simulink model "aeromissile_la"  (R2019b)
settings: Solver=ode45  StartTime=0.0  StopTime=20  RelTol=1e-3  EnableMultiTasking=on
PreLoadFcn:
  | aeromissile_la_dat
values from neighbouring files (symbols this model uses):
  cy_el = 0.034000/d2r    (= 1.94805650344)    [aeromissile_la_dat.m]
  cz_el = -0.034000/d2r    (= -1.94805650344)    [aeromissile_la_dat.m]
  d_ref = 0.2286    [aeromissile_la_dat.m]
  eul_0 = [0;0;0]    [aeromissile_la_dat.m]
  fin_max = 30.0*d2r    (= 0.523598775598)    [aeromissile_la_dat.m]
  fin_min = -30.0*d2r    (= -0.523598775598)    [aeromissile_la_dat.m]
  g = 9.81    [aeromissile_la_dat.m]
  inertia = inertia_0/2    [aeromissile_la_dat.m]
  inertia_0 = diag([Ixx Iyy Izz])    [aeromissile_la_dat.m]
  l_acc = 0.5    [aeromissile_la_dat.m]
  l_ref = 0.04    [aeromissile_la_dat.m]
  len_missile = 3    [aeromissile_la_dat.m]
  mass_0 = 234.02    [aeromissile_la_dat.m]
  massf = 30    [aeromissile_la_dat.m]
  mx_el = -0.206000/d2r    (= -11.8029305797)    [aeromissile_la_dat.m]
  mx_wx = -0.5    [aeromissile_la_dat.m]
  my_el = -0.206000/d2r    (= -11.8029305797)    [aeromissile_la_dat.m]
  my_wy = -1.719    [aeromissile_la_dat.m]
  mz_el = -0.206000/d2r    (= -11.8029305797)    [aeromissile_la_dat.m]
  mz_wz = -1.719    [aeromissile_la_dat.m]
  q = 2    [aeromissile_la_dat.m]
  S_ref = 0.040877    [aeromissile_la_dat.m]
  Thrust = 10e3    (= 10000)    [aeromissile_la_dat.m]
  Vm_0 = [300;0;0]    [aeromissile_la_dat.m]
  wm_0 = [0;0;0]    [aeromissile_la_dat.m]
  x_cg = 0.555*len_missile    (= 1.665)    [aeromissile_la_dat.m]
  x_cg_0 = 0.575*len_missile    (= 1.725)    [aeromissile_la_dat.m]
  x_ref = 0.54*len_missile    (= 1.62)    [aeromissile_la_dat.m]
  xmg_0 = [0;1000;0]    [aeromissile_la_dat.m]
undefined symbols (not defined in the file or in its folder): Earth, inv_fcn, WGS84
libraries: simulink_need_slupdate x26, sharedutil x3, aerolibobsolete x2, aerolibtransform2 x2, aerolibfltsims x2, aerolibprivatev1p5 x1, vrlib x1
(part 2 of 2)

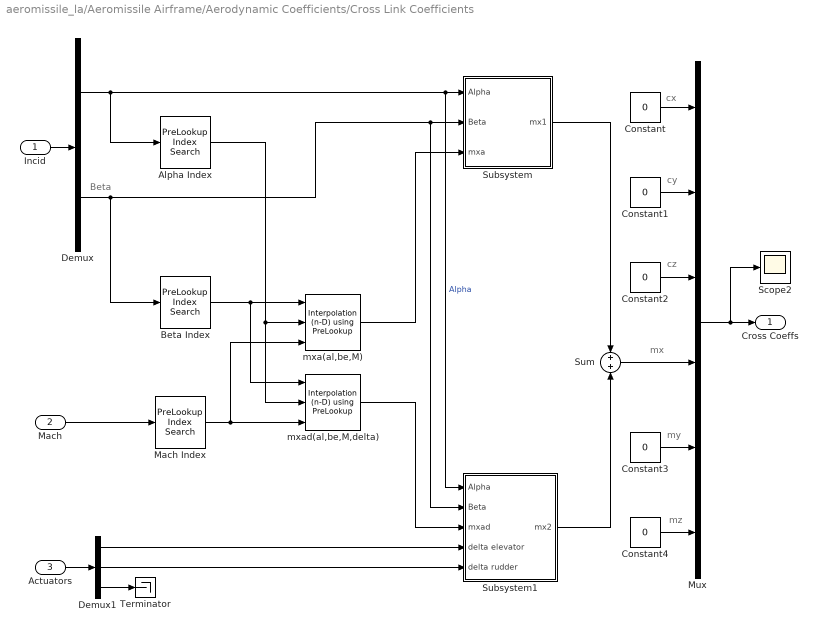
== system aeromissile_la/Aeromissile Airframe/Aerodynamic Coefficients/Cross Link Coefficients ==
  note: Beta
  note: cy
  note: cx
  note: cz
  note: mx
  note: my
  note: mz
  Incid : Inport
  Mach : Inport  Port=2
  Actuators : Inport  Port=3
  Alpha Index : simulink_need_slupdate/PreLookup Index Search  bpData=alpha_vec  searchMode=Binary Search  cacheBpFlag=on  outputFlag=off  IndexDataType=uint32  extrapMode=Linear Extrapolation  rangeErrorMode=None
      settings: SourceProductName=Simulink  SourceProductBaseCode=SL
  Beta Index : simulink_need_slupdate/PreLookup Index Search  bpData=beta_vec  searchMode=Binary Search  cacheBpFlag=on  outputFlag=off  IndexDataType=uint32  extrapMode=Linear Extrapolation  rangeErrorMode=None
      settings: SourceProductName=Simulink  SourceProductBaseCode=SL
  Constant{,1..4} (5 alike) : Constant  Value=0
  Demux : Demux  Outputs=2
  Demux1 : Demux  Outputs=3
  Mach Index : simulink_need_slupdate/PreLookup Index Search  bpData=Mach_vec  searchMode=Binary Search  cacheBpFlag=on  outputFlag=off  IndexDataType=uint32  extrapMode=Linear Extrapolation  rangeErrorMode=None
      settings: SourceProductName=Simulink  SourceProductBaseCode=SL
  Mux : Mux  Inputs=6
  Scope2 : Scope
  Subsystem : Subsystem
  Subsystem1 : Subsystem
  Sum : Sum  SaturateOnIntegerOverflow=on
  Terminator : Terminator
  mxa(al,be,M) : simulink_need_slupdate/Interpolation (n-D) using PreLookup  numDimsPopupSelect=3  explicitNumDims=2  table=mxa  interpMethod=Linear  extrapMethod=Linear  rangeErrorMode=None  NumSelectionDims=0
      settings: SourceProductName=Simulink  SourceProductBaseCode=SL
  mxad(al,be,M,delta) : simulink_need_slupdate/Interpolation (n-D) using PreLookup  numDimsPopupSelect=3  explicitNumDims=2  table=mxad  interpMethod=Linear  extrapMethod=Linear  rangeErrorMode=None  NumSelectionDims=0
      settings: SourceProductName=Simulink  SourceProductBaseCode=SL
  Cross Coeffs : Outport  InitialOutput=0
  wires:
  Mach/1 -> Mach Index/1
  Demux/1 -> Alpha Index/1, Subsystem/1(Alpha), Subsystem1/1(Alpha)  "Alpha"
  Demux/2 -> Beta Index/1, Subsystem/2(Beta), Subsystem1/2(Beta)
  Incid/1 -> Demux/1
  Constant/1 -> Mux/1
  Constant1/1 -> Mux/2
  Constant2/1 -> Mux/3
  Constant3/1 -> Mux/5
  Constant4/1 -> Mux/6
  Mux/1 -> Cross Coeffs/1, Scope2/1
  Alpha Index/1 -> mxa(al,be,M)/2, mxad(al,be,M,delta)/2
  Beta Index/1 -> mxa(al,be,M)/1, mxad(al,be,M,delta)/1
  Mach Index/1 -> mxad(al,be,M,delta)/3, mxa(al,be,M)/3
  Actuators/1 -> Demux1/1
  Demux1/1 -> Subsystem1/4(delta elevator)
  Demux1/2 -> Subsystem1/5(delta rudder)
  Demux1/3 -> Terminator/1
  Sum/1 -> Mux/4
  Subsystem/1(mx1) -> Sum/1
  mxa(al,be,M)/1 -> Subsystem/3(mxa)
  mxad(al,be,M,delta)/1 -> Subsystem1/3(mxad)
  Subsystem1/1(mx2) -> Sum/2

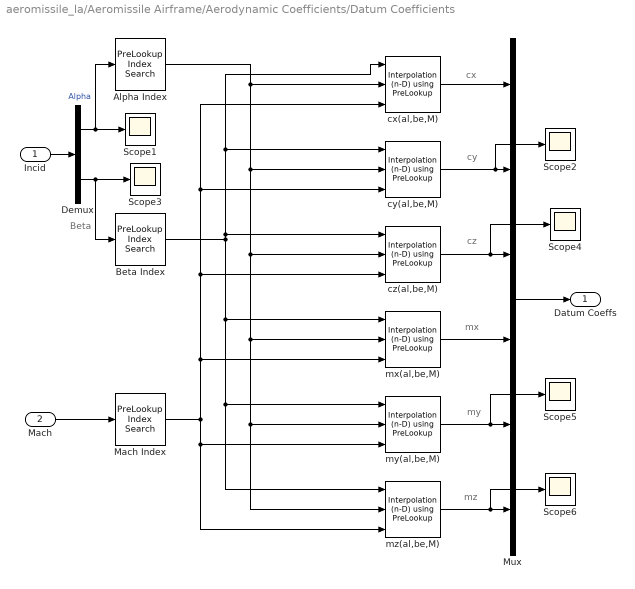
== system aeromissile_la/Aeromissile Airframe/Aerodynamic Coefficients/Datum Coefficients ==
  note: Beta
  note: cy
  note: cx
  note: cz
  note: mx
  note: my
  note: mz
  Incid : Inport
  Mach : Inport  Port=2
  Alpha Index : simulink_need_slupdate/PreLookup Index Search  bpData=alpha_vec  searchMode=Binary Search  cacheBpFlag=on  outputFlag=off  IndexDataType=uint32  extrapMode=Linear Extrapolation  rangeErrorMode=None
      settings: SourceProductName=Simulink  SourceProductBaseCode=SL
  Beta Index : simulink_need_slupdate/PreLookup Index Search  bpData=beta_vec  searchMode=Binary Search  cacheBpFlag=on  outputFlag=off  IndexDataType=uint32  extrapMode=Linear Extrapolation  rangeErrorMode=None
      settings: SourceProductName=Simulink  SourceProductBaseCode=SL
  Demux : Demux  Outputs=2
  Mach Index : simulink_need_slupdate/PreLookup Index Search  bpData=Mach_vec  searchMode=Binary Search  cacheBpFlag=on  outputFlag=off  IndexDataType=uint32  extrapMode=Linear Extrapolation  rangeErrorMode=None
      settings: SourceProductName=Simulink  SourceProductBaseCode=SL
  Mux : Mux  Inputs=6
  Scope{1..6} (6 alike) : Scope
  cx(al,be,M) : simulink_need_slupdate/Interpolation (n-D) using PreLookup  numDimsPopupSelect=3  explicitNumDims=2  table=cx  interpMethod=Linear  extrapMethod=Linear  rangeErrorMode=None  NumSelectionDims=0
      settings: SourceProductName=Simulink  SourceProductBaseCode=SL
  cy(al,be,M) : simulink_need_slupdate/Interpolation (n-D) using PreLookup  numDimsPopupSelect=3  explicitNumDims=2  table=cy  interpMethod=Linear  extrapMethod=Linear  rangeErrorMode=None  NumSelectionDims=0
      settings: SourceProductName=Simulink  SourceProductBaseCode=SL
  cz(al,be,M) : simulink_need_slupdate/Interpolation (n-D) using PreLookup  numDimsPopupSelect=3  explicitNumDims=2  table=cz  interpMethod=Linear  extrapMethod=Linear  rangeErrorMode=None  NumSelectionDims=0
      settings: SourceProductName=Simulink  SourceProductBaseCode=SL
  mx(al,be,M) : simulink_need_slupdate/Interpolation (n-D) using PreLookup  numDimsPopupSelect=3  explicitNumDims=2  table=mx  interpMethod=Linear  extrapMethod=Linear  rangeErrorMode=None  NumSelectionDims=0
      settings: SourceProductName=Simulink  SourceProductBaseCode=SL
  my(al,be,M) : simulink_need_slupdate/Interpolation (n-D) using PreLookup  numDimsPopupSelect=3  explicitNumDims=2  table=my  interpMethod=Linear  extrapMethod=Linear  rangeErrorMode=None  NumSelectionDims=0
      settings: SourceProductName=Simulink  SourceProductBaseCode=SL
  mz(al,be,M) : simulink_need_slupdate/Interpolation (n-D) using PreLookup  numDimsPopupSelect=3  explicitNumDims=2  table=mz  interpMethod=Linear  extrapMethod=Linear  rangeErrorMode=None  NumSelectionDims=0
      settings: SourceProductName=Simulink  SourceProductBaseCode=SL
  Datum Coeffs : Outport  InitialOutput=0
  wires:
  Alpha Index/1 -> my(al,be,M)/2, mz(al,be,M)/2, mx(al,be,M)/2, cz(al,be,M)/2, cy(al,be,M)/2, cx(al,be,M)/2
  Mach Index/1 -> cx(al,be,M)/3, cy(al,be,M)/3, cz(al,be,M)/3, my(al,be,M)/3, mz(al,be,M)/3, mx(al,be,M)/3
  Mach/1 -> Mach Index/1
  Beta Index/1 -> cx(al,be,M)/1, cy(al,be,M)/1, my(al,be,M)/1, mz(al,be,M)/1, mx(al,be,M)/1, cz(al,be,M)/1
  Demux/1 -> Alpha Index/1, Scope1/1  "Alpha"
  Demux/2 -> Beta Index/1, Scope3/1
  Incid/1 -> Demux/1
  cx(al,be,M)/1 -> Mux/1
  cy(al,be,M)/1 -> Mux/2, Scope2/1
  cz(al,be,M)/1 -> Mux/3, Scope4/1
  mx(al,be,M)/1 -> Mux/4
  my(al,be,M)/1 -> Mux/5, Scope5/1
  mz(al,be,M)/1 -> Mux/6, Scope6/1
  Mux/1 -> Datum Coeffs/1

== system aeromissile_la/Aeromissile Airframe/Aerodynamic Forces and Moments/Moments about Centre of Gravity ==
  Clock : Clock
  Constant1 : Constant  Value=massf
  Constant2 : Constant  Value=q
  Constant4 : Constant  Value=x_ref
  Constant5 : Constant  Value=x_cg_0
  Constant6 : Constant  Value=x_cg_0
  Constant7 : Constant  Value=x_cg
  Constant8 : Constant  Value=0
  Constant9 : Constant  Value=x_cg
  Gain1 : Gain  Gain=-1  SaturateOnIntegerOverflow=on  OutDataTypeStr=Inherit: Same as input  ParamDataTypeStr=Inherit: Same as input
  Mux : Mux  Inputs=3
  Product1 : Product  SaturateOnIntegerOverflow=on  OutDataTypeStr=Inherit: Same as first input
  Product2 : Product  Inputs=**/*  SaturateOnIntegerOverflow=on  OutDataTypeStr=Inherit: Same as first input
  Sum{2..5} (4 alike) : Sum  Inputs=|+-  SaturateOnIntegerOverflow=on
  Switch : Switch  Criteria=u2 > Threshold  SaturateOnIntegerOverflow=on
  -(x_cg-x_ref) : Outport
  tag scope: x_cg_t=global
  wires:
  Clock/1 -> Product1/2, Product2/4
  Constant1/1 -> Sum2/1, Product2/3
  Product1/1 -> Sum2/2
  Sum2/1 -> Switch/2
  Constant5/1 -> Sum3/1
  Constant6/1 -> Sum4/1
  Constant7/1 -> Sum4/2
  Product2/1 -> Sum3/2
  Sum3/1 -> Switch/1
  Constant9/1 -> Switch/3
  Switch/1 -> Sum5/1, [x_cg_t]
  Constant4/1 -> Sum5/2
  Sum5/1 -> Gain1/1
  Gain1/1 -> Mux/1
  Mux/1 -> -(x_cg-x_ref)/1
  Constant8/1 -> Mux/3, Mux/2
  Constant2/1 -> Product1/1, Product2/2
  Sum4/1 -> Product2/1

== system aeromissile_la/Aeromissile Airframe/Environment Models/Wind Models ==
  Altitude : Inport
  DCM : Inport  Port=2
  Airspeed : Inport  Port=3
  Constant : Constant  Value=[0 0 0]
  Constant1 : Constant  Value=[0 0 0]
  Terminator{,1..4} (5 alike) : Terminator
  ux,uy,uz : Outport
  wux,wuy,wuz : Outport  Port=2
  wires:
  Altitude/1 -> Terminator2/1, Terminator/1
  DCM/1 -> Terminator1/1
  Airspeed/1 -> Terminator3/1, Terminator4/1
  Constant1/1 -> wux,wuy,wuz/1
  Constant/1 -> ux,uy,uz/1

== system aeromissile_la/Aeromissile Airframe/Environment Models/m(t) ==
  Clock : Clock
  Constant : Constant  Value=mass_0
  Constant1 : Constant  Value=massf
  Constant2 : Constant  Value=q
  Product : Product  SaturateOnIntegerOverflow=on  OutDataTypeStr=Inherit: Same as first input
  Scope : Scope
  Sum2 : Sum  Inputs=|+-  SaturateOnIntegerOverflow=on
  Sum4 : Sum  Inputs=|+-  SaturateOnIntegerOverflow=on
  Sum5 : Sum  Inputs=|+-  SaturateOnIntegerOverflow=on
  Switch1 : Switch  Criteria=u2 > Threshold  SaturateOnIntegerOverflow=on
  m(t) : Outport
  wires:
  Constant2/1 -> Product/1
  Clock/1 -> Product/2
  Constant1/1 -> Sum2/1, Sum4/2
  Product/1 -> Sum2/2, Sum5/2
  Sum2/1 -> Switch1/2
  Sum4/1 -> Switch1/3
  Constant/1 -> Sum5/1, Sum4/1
  Sum5/1 -> Switch1/1
  Switch1/1 -> Scope/1, m(t)/1  "m(t)"

== system aeromissile_la/Aeromissile Airframe/Flight LA/FlightGear Animation LA ==
  Xg : Inport
  Euler : Inport  Port=2
  -h_1 : Constant  Value=-1000
  Demux3 : Demux  Outputs=2
  Demux4 : Demux  Outputs=3
  Demux5 : Demux  Outputs=3
  Flat Earth to LLA1 : aerolibtransform2/Flat Earth to LLA  units=Metric (MKS)  ptype=Earth (WGS84)  F=1/298.257223563  R=6378137  LL0=[0 0]  psi=0
  FlightGear Preconfigured 6DoF Animation LA : aerolibfltsims/FlightGear Preconfigured 6DoF Animation  xFlightGearVersion=v2018.3  DestinationIpAddress=127.0.0.1  DestinationPort=5004  SampleTime=1/60  packetVersion=24
      settings: SourceProductName=Aerospace Blockset
  Mux2 : Mux  Inputs=6
  Mux3 : Mux  Inputs=3
  Unary Minus2 : UnaryMinus
  wires:
  Flat Earth to LLA1/1 -> Demux3/1
  Unary Minus2/1 -> Mux3/3
  Demux5/2 -> Unary Minus2/1
  -h_1/1 -> Flat Earth to LLA1/2
  Demux5/1 -> Mux3/1
  Mux3/1 -> Flat Earth to LLA1/1
  Flat Earth to LLA1/2 -> Mux2/3
  Demux4/1 -> Mux2/4  "phi"
  Demux4/3 -> Mux2/6  "psi"
  Demux5/3 -> Mux3/2
  Demux4/2 -> Mux2/5  "theta"
  Demux3/1 -> Mux2/2
  Demux3/2 -> Mux2/1
  Mux2/1 -> FlightGear Preconfigured 6DoF Animation LA/1
  Euler/1 -> Demux4/1
  Xg/1 -> Demux5/1

== system aeromissile_la/Aeromissile Airframe/Start Init/Subsystem ==
  Vg_m : Inport
  Vg_la : Inport  Port=2
  Switch3 : Switch  Criteria=u2 ~= 0  SaturateOnIntegerOverflow=on
  Vg : Outport
  wires:
  Switch3/1 -> Vg/1
  Vg_m/1 -> Switch3/1
  Vg_la/1 -> Switch3/3
  [Start] -> Switch3/2

== system aeromissile_la/Aeromissile Airframe/Start Init/Subsystem1 ==
  Xg_m : Inport
  Xg_la : Inport  Port=2
  Switch3 : Switch  Criteria=u2 ~= 0  SaturateOnIntegerOverflow=on
  "Xg " : Outport
  wires:
  Switch3/1 -> "Xg "/1
  Xg_m/1 -> Switch3/1
  Xg_la/1 -> Switch3/3
  [Start] -> Switch3/2

== system aeromissile_la/Aeromissile Airframe/Start Init/Subsystem2 ==
  DCM_m : Inport
  DCM_la : Inport  Port=2
  Reshape 1x9->3x3 : Reshape  OutputDimensionality=Customize  OutputDimensions=[3,3]
  Reshape 3x3->1x9 : Reshape  OutputDimensionality=Customize  OutputDimensions=[1,9]
  "Reshape 3x3->1x9 " : Reshape  OutputDimensionality=Customize  OutputDimensions=[1,9]
  Switch : Switch  Criteria=u2 ~= 0  SaturateOnIntegerOverflow=on
  "DCM " : Outport
  wires:
  DCM_m/1 -> Reshape 3x3->1x9/1
  DCM_la/1 -> "Reshape 3x3->1x9 "/1
  Reshape 3x3->1x9/1 -> Switch/1
  "Reshape 3x3->1x9 "/1 -> Switch/3
  Reshape 1x9->3x3/1 -> "DCM "/1
  Switch/1 -> Reshape 1x9->3x3/1
  [Start] -> Switch/2

== system aeromissile_la/Aeromissile Airframe/Start Init/Subsystem3 ==
  w_m : Inport
  w_la : Inport  Port=2
  Switch3 : Switch  Criteria=u2 ~= 0  SaturateOnIntegerOverflow=on
  "w " : Outport
  wires:
  Switch3/1 -> "w "/1
  w_m/1 -> Switch3/1
  w_la/1 -> Switch3/3
  [Start] -> Switch3/2

== system aeromissile_la/Aeromissile Airframe/Start Init/Subsystem4 ==
  dw/dt_m : Inport
  dw/dt_la : Inport  Port=2
  Switch3 : Switch  Criteria=u2 ~= 0  SaturateOnIntegerOverflow=on
  "dw/dt " : Outport
  wires:
  Switch3/1 -> "dw/dt "/1
  dw/dt_m/1 -> Switch3/1
  dw/dt_la/1 -> Switch3/3
  [Start] -> Switch3/2

== system aeromissile_la/Aeromissile Airframe/Start Init/Subsystem5 ==
  Accels_m : Inport
  Accels_la : Inport  Port=2
  Switch3 : Switch  Criteria=u2 ~= 0  SaturateOnIntegerOverflow=on
  "Accels " : Outport
  wires:
  Switch3/1 -> "Accels "/1
  Accels_m/1 -> Switch3/1
  Accels_la/1 -> Switch3/3
  [Start] -> Switch3/2

== system aeromissile_la/Aeromissile Airframe/Start Init/Subsystem6 ==
  Incid_m : Inport
  Incid_la : Inport  Port=2
  Switch3 : Switch  Criteria=u2 ~= 0  SaturateOnIntegerOverflow=on
  "Incid " : Outport
  wires:
  Switch3/1 -> "Incid "/1
  Incid_m/1 -> Switch3/1
  Incid_la/1 -> Switch3/3
  [Start] -> Switch3/2

== system aeromissile_la/Aeromissile Airframe/Start Init/Subsystem7 ==
  Euler_m : Inport
  Euler_la : Inport  Port=2
  Switch3 : Switch  Criteria=u2 ~= 0  SaturateOnIntegerOverflow=on
  "Euler " : Outport
  wires:
  Switch3/1 -> "Euler "/1
  Euler_m/1 -> Switch3/1
  Euler_la/1 -> Switch3/3
  [Start] -> Switch3/2

== system aeromissile_la/Aeromissile Airframe/Start Init/Subsystem8 ==
  Vc_m : Inport
  Vc_la : Inport  Port=2
  Switch3 : Switch  Criteria=u2 ~= 0  SaturateOnIntegerOverflow=on
  "Vc " : Outport
  wires:
  Switch3/1 -> "Vc "/1
  Vc_m/1 -> Switch3/1
  Vc_la/1 -> Switch3/3
  [Start] -> Switch3/2

== system aeromissile_la/Aeromissile Airframe/Start Init/Subsystem9 ==
  M_q_m : Inport
  M_q_la : Inport  Port=2
  Switch3 : Switch  Criteria=u2 ~= 0  SaturateOnIntegerOverflow=on
  "M_q " : Outport
  wires:
  Switch3/1 -> "M_q "/1
  M_q_m/1 -> Switch3/1
  M_q_la/1 -> Switch3/3
  [Start] -> Switch3/2

== system aeromissile_la/Aeromissile Airframe/Thrust(t)/Subsystem ==
  Actuators : Inport
  Constant6 : Constant  Value=Thrust
  Demux1 : Demux  Outputs=3
  Gain : Gain  Gain=-1  SaturateOnIntegerOverflow=on  OutDataTypeStr=Inherit: Same as input  ParamDataTypeStr=Inherit: Same as input
  Mux1 : Mux  Inputs=3
  Product1 : Product  Inputs=3  SaturateOnIntegerOverflow=on  OutDataTypeStr=Inherit: Same as first input
  Product2 : Product  SaturateOnIntegerOverflow=on  OutDataTypeStr=Inherit: Same as first input
  Product3 : Product  SaturateOnIntegerOverflow=on  OutDataTypeStr=Inherit: Same as first input
  Scope2 : Scope
  Terminator : Terminator
  Trigonometric Function : Trigonometry  Operator=cos
  Trigonometric Function1 : Trigonometry  Operator=cos
  Trigonometric Function2 : Trigonometry
  Trigonometric Function3 : Trigonometry
  if |u|<0.1 : Subsystem
  "if |u|<0.1 " : Subsystem
  Thrust : Outport
  wires:
  Constant6/1 -> Product1/1, Product2/1, Product3/1
  Trigonometric Function/1 -> Product1/2
  Trigonometric Function1/1 -> Product1/3
  Product1/1 -> Mux1/1  "Tx"
  Trigonometric Function2/1 -> Product2/2
  Product2/1 -> Mux1/2  "Ty"
  Product3/1 -> Mux1/3  "Tz"
  Trigonometric Function3/1 -> Product3/2
  Actuators/1 -> Demux1/1
  Gain/1 -> Trigonometric Function3/1
  Demux1/2 -> "if |u|<0.1 "/1(in)  "rudder actuators"
  Demux1/3 -> Terminator/1
  Mux1/1 -> Thrust/1, Scope2/1
  Demux1/1 -> if |u|<0.1/1(in)  "elevator actuators"
  if |u|<0.1/1(out) -> Trigonometric Function/1, Trigonometric Function2/1
  "if |u|<0.1 "/1(out) -> Trigonometric Function1/1, Gain/1

== system aeromissile_la/Autopilot/Pitch Autopilot/Gain Scheduled Coefficients Alpha ==
  Alpha : Inport
  Mach : Inport  Port=2
  Abs : Abs  SaturateOnIntegerOverflow=on
  K : simulink_need_slupdate/Interpolation (n-D) using PreLookup  numDimsPopupSelect=2  explicitNumDims=2  table=K  interpMethod=Linear  extrapMethod=Linear  rangeErrorMode=None  NumSelectionDims=0
      settings: SourceProductName=Simulink  SourceProductBaseCode=SL
  Ka : simulink_need_slupdate/Interpolation (n-D) using PreLookup  numDimsPopupSelect=2  explicitNumDims=2  table=Ka  interpMethod=Linear  extrapMethod=Linear  rangeErrorMode=None  NumSelectionDims=0
      settings: SourceProductName=Simulink  SourceProductBaseCode=SL
  Kg : simulink_need_slupdate/Interpolation (n-D) using PreLookup  numDimsPopupSelect=2  explicitNumDims=2  table=Kg  interpMethod=Linear  extrapMethod=Linear  rangeErrorMode=None  NumSelectionDims=0
      settings: SourceProductName=Simulink  SourceProductBaseCode=SL
  Ki : simulink_need_slupdate/Interpolation (n-D) using PreLookup  numDimsPopupSelect=2  explicitNumDims=2  table=Ki  interpMethod=Linear  extrapMethod=Linear  rangeErrorMode=None  NumSelectionDims=0
      settings: SourceProductName=Simulink  SourceProductBaseCode=SL
  Mach Index : simulink_need_slupdate/PreLookup Index Search  bpData=M_sch  searchMode=Binary Search  cacheBpFlag=on  outputFlag=off  IndexDataType=uint32  extrapMode=Linear Extrapolation  rangeErrorMode=None
      settings: SourceProductName=Simulink  SourceProductBaseCode=SL
  |Alpha| Index : simulink_need_slupdate/PreLookup Index Search  bpData=alpha_sch  searchMode=Binary Search  cacheBpFlag=on  outputFlag=off  IndexDataType=uint32  extrapMode=Linear Extrapolation  rangeErrorMode=None
      settings: SourceProductName=Simulink  SourceProductBaseCode=SL
  "Kg " : Outport  InitialOutput=0
  "KI " : Outport  Port=2  InitialOutput=0
  "K " : Outport  Port=3  InitialOutput=0
  "Ka " : Outport  Port=4  InitialOutput=0
  wires:
  Mach Index/1 -> Ka/1, K/1, Ki/1, Kg/1
  |Alpha| Index/1 -> Ka/2, K/2, Ki/2, Kg/2
  Ka/1 -> "Ka "/1
  K/1 -> "K "/1
  Ki/1 -> "KI "/1
  Kg/1 -> "Kg "/1
  Abs/1 -> |Alpha| Index/1
  Mach/1 -> Mach Index/1
  Alpha/1 -> Abs/1

== system aeromissile_la/Autopilot/Yaw Autopilot/Gain Scheduled Coefficients Beta ==
  Beta : Inport
  Mach : Inport  Port=2
  Abs : Abs  SaturateOnIntegerOverflow=on
  K : simulink_need_slupdate/Interpolation (n-D) using PreLookup  numDimsPopupSelect=2  explicitNumDims=2  table=K  interpMethod=Linear  extrapMethod=Linear  rangeErrorMode=None  NumSelectionDims=0
      settings: SourceProductName=Simulink  SourceProductBaseCode=SL
  Ka : simulink_need_slupdate/Interpolation (n-D) using PreLookup  numDimsPopupSelect=2  explicitNumDims=2  table=Ka  interpMethod=Linear  extrapMethod=Linear  rangeErrorMode=None  NumSelectionDims=0
      settings: SourceProductName=Simulink  SourceProductBaseCode=SL
  Kg : simulink_need_slupdate/Interpolation (n-D) using PreLookup  numDimsPopupSelect=2  explicitNumDims=2  table=Kg  interpMethod=Linear  extrapMethod=Linear  rangeErrorMode=None  NumSelectionDims=0
      settings: SourceProductName=Simulink  SourceProductBaseCode=SL
  Ki : simulink_need_slupdate/Interpolation (n-D) using PreLookup  numDimsPopupSelect=2  explicitNumDims=2  table=Ki  interpMethod=Linear  extrapMethod=Linear  rangeErrorMode=None  NumSelectionDims=0
      settings: SourceProductName=Simulink  SourceProductBaseCode=SL
  Mach Index : simulink_need_slupdate/PreLookup Index Search  bpData=M_sch  searchMode=Binary Search  cacheBpFlag=on  outputFlag=off  IndexDataType=uint32  extrapMode=Linear Extrapolation  rangeErrorMode=None
      settings: SourceProductName=Simulink  SourceProductBaseCode=SL
  |Beta| Index : simulink_need_slupdate/PreLookup Index Search  bpData=alpha_sch  searchMode=Binary Search  cacheBpFlag=on  outputFlag=off  IndexDataType=uint32  extrapMode=Linear Extrapolation  rangeErrorMode=None
      settings: SourceProductName=Simulink  SourceProductBaseCode=SL
  "Kg " : Outport  InitialOutput=0
  "KI " : Outport  Port=2  InitialOutput=0
  "K " : Outport  Port=3  InitialOutput=0
  "Ka " : Outport  Port=4  InitialOutput=0
  wires:
  Mach Index/1 -> Ka/1, K/1, Ki/1, Kg/1
  |Beta| Index/1 -> Ka/2, K/2, Ki/2, Kg/2
  Ka/1 -> "Ka "/1
  K/1 -> "K "/1
  Ki/1 -> "KI "/1
  Kg/1 -> "Kg "/1
  Abs/1 -> |Beta| Index/1
  Mach/1 -> Mach Index/1
  Beta/1 -> Abs/1

== system aeromissile_la/Start Time/t departure/If Action Subsystem ==
  In1 : Inport
  Action Port : ActionPort  ActionPortLabel=if(u1 <= 1.5)
  Out1 : Outport
  wires:
  In1/1 -> Out1/1

== system aeromissile_la/Start Time/t engine/If Action Subsystem1 ==
  In1 : Inport
  Action Port : ActionPort  ActionPortLabel=if(u1 <= 3)
  Out1 : Outport
  wires:
  In1/1 -> Out1/1

== system aeromissile_la/Start Time/t start/If Action Subsystem ==
  In1 : Inport
  Action Port : ActionPort  ActionPortLabel=if(u1 == 0)
  Out1 : Outport
  wires:
  In1/1 -> Out1/1

== system aeromissile_la/Visualisation/VR Sink Animation/Euler to VR Quaternion ==
  Euler Angles : Inport
  .... followed by Yaw : Subsystem  mask(Quaternion product){}
      mask help: Perform quaternion multiplication e1*e0, where e0 is the first rotation and e1 is the second rotation.
  "Align object " : Subsystem  mask(Quaternion product){}
      mask help: Perform quaternion multiplication e1*e0, where e0 is the first rotation and e1 is the second rotation.
  Demux : Demux  Outputs=3
  Initial Roll by 90 degrees : Constant  Value=pi/2
  Mux{,1..3} (4 alike) : Mux  Inputs=2
  Quaternion Normalisation : Subsystem
  "Quaternion Normalisation " : Subsystem
  "Quaternion Normalisation  " : Subsystem
  "Quaternion Normalisation   " : Subsystem
  Quaternion Vector : Subsystem
  Roll followed by Pitch : Subsystem  mask(Quaternion product){}
      mask help: Perform quaternion multiplication e1*e0, where e0 is the first rotation and e1 is the second rotation.
  Vr Pitch : Constant  Value=[0 0 1]
  Vr Pitch Axes : Constant  Value=[0 0 1]
  Vr Roll Axes : Constant  Value=[1 0 0]
  Vr Yaw Axes : Constant  Value=[0 1 0]
  Quaternion : Outport
  wires:
  Mux3/1 -> "Quaternion Normalisation "/1(e0)
  Initial Roll by 90 degrees/1 -> Mux3/2
  Vr Pitch/1 -> Mux3/1
  Mux2/1 -> "Quaternion Normalisation   "/1(e0)
  Mux1/1 -> "Quaternion Normalisation  "/1(e0)
  Mux/1 -> Quaternion Normalisation/1(e0)
  Demux/3 -> Mux2/2
  Vr Yaw Axes/1 -> Mux2/1
  Demux/2 -> Mux1/2
  Vr Pitch Axes/1 -> Mux1/1
  Demux/1 -> Mux/2
  Vr Roll Axes/1 -> Mux/1
  Euler Angles/1 -> Demux/1
  .... followed by Yaw/1(e3) -> Quaternion Vector/1(e0)
  Quaternion Vector/1(e0_norm) -> Quaternion/1
  "Quaternion Normalisation "/1(e0_norm) -> "Align object "/1(e0)
  Quaternion Normalisation/1(e0_norm) -> "Align object "/2("e1 ")
  "Quaternion Normalisation  "/1(e0_norm) -> Roll followed by Pitch/2("e1 ")
  "Align object "/1(e3) -> Roll followed by Pitch/1(e0)
  "Quaternion Normalisation   "/1(e0_norm) -> .... followed by Yaw/2("e1 ")
  Roll followed by Pitch/1(e3) -> .... followed by Yaw/1(e0)

== system aeromissile_la/Aeromissile Airframe/6DoF Ru (Euler Angles) Mvar/inertia^(-1)x(M-C)/inertia(t)^-1 ==
  Scope : Scope
  Scope1 : Scope
  inertia(t) : Subsystem
  inv_fcn : MATLABFcn  MATLABFcn=inv_fcn(u)  OutputDimensions=[3 3]  Output1D=off
  inertia(t)^-1 : Outport
  wires:
  inertia(t)/1(inertia(t)) -> inv_fcn/1, Scope1/1
  inv_fcn/1 -> inertia(t)^-1/1, Scope/1

== system aeromissile_la/Aeromissile Airframe/6DoF Ru (Euler Angles) Mvar/inertiaxw/inertia(t) ==
  Constant : Constant  Value=inertia_0
  Constant1 : Constant  Value=inertia
  Constant2 : Constant  Value=q
  Constant3 : Constant  Value=massf
  Product : Product  Inputs=**/  SaturateOnIntegerOverflow=on  OutDataTypeStr=Inherit: Same as first input
  Product1 : Product  SaturateOnIntegerOverflow=on  OutDataTypeStr=Inherit: Same as first input
  Scope : Scope
  Sum : Sum  Inputs=|+-  SaturateOnIntegerOverflow=on
  Sum1 : Sum  Inputs=|+-  SaturateOnIntegerOverflow=on
  Sum3 : Sum  Inputs=|+-  SaturateOnIntegerOverflow=on
  Switch : Switch  Criteria=u2 > Threshold  SaturateOnIntegerOverflow=on
  inertia(t) : Outport
  wires:
  Constant/1 -> Sum1/1, Sum/1
  Constant1/1 -> Sum1/2, Switch/3
  Sum1/1 -> Product/1
  Product/1 -> Sum/2
  Switch/1 -> inertia(t)/1, Scope/1
  Sum/1 -> Switch/1
  Constant2/1 -> Product1/1
  [tE] -> Product1/2
  Sum3/1 -> Switch/2
  Product1/1 -> Product/2, Sum3/2
  Constant3/1 -> Product/3, Sum3/1

== system aeromissile_la/Aeromissile Airframe/Aerodynamic Coefficients/Cross Link Coefficients/Subsystem ==
  Alpha : Inport
  Beta : Inport  Port=2
  mxa : Inport  Port=3
  Constant1 : Constant  Value=0.0001
  Constant5 : Constant  Value=4
  Gain : Gain  Gain=-1  SaturateOnIntegerOverflow=on  OutDataTypeStr=Inherit: Same as input  ParamDataTypeStr=Inherit: Same as input
  Math Function : Math  Operator=square  SaturateOnIntegerOverflow=on
  Math Function1 : Math  Operator=square  SaturateOnIntegerOverflow=on
  Product1 : Product  Inputs=****/*  SaturateOnIntegerOverflow=on  OutDataTypeStr=Inherit: Same as first input
  Sum1 : Sum  Inputs=-+  SaturateOnIntegerOverflow=on
  Sum2 : Sum  SaturateOnIntegerOverflow=on
  Switch : Switch  Criteria=u2 ~= 0  SaturateOnIntegerOverflow=on
  mx1 : Outport
  wires:
  Gain/1 -> Product1/3
  Math Function1/1 -> Sum1/2, Sum2/2
  Math Function/1 -> Sum1/1, Sum2/1
  Constant5/1 -> Product1/4
  Alpha/1 -> Math Function/1, Product1/2
  Beta/1 -> Gain/1, Math Function1/1
  Sum1/1 -> Product1/1
  Sum2/1 -> Switch/2, Switch/1
  Product1/1 -> mx1/1
  Switch/1 -> Product1/5
  mxa/1 -> Product1/6
  Constant1/1 -> Switch/3

== system aeromissile_la/Aeromissile Airframe/Aerodynamic Coefficients/Cross Link Coefficients/Subsystem1 ==
  Alpha : Inport
  Beta : Inport  Port=2
  mxad : Inport  Port=3
  delta elevator : Inport  Port=4
  delta rudder : Inport  Port=5
  Constant1 : Constant  Value=0.0001
  Constant5 : Constant  Value=0.0352
  Gain : Gain  Gain=-1  SaturateOnIntegerOverflow=on  OutDataTypeStr=Inherit: Same as input  ParamDataTypeStr=Inherit: Same as input
  Gain1 : Gain  Gain=-1  SaturateOnIntegerOverflow=on  OutDataTypeStr=Inherit: Same as input  ParamDataTypeStr=Inherit: Same as input
  Math Function : Math  Operator=square  SaturateOnIntegerOverflow=on
  Math Function1 : Math  Operator=square  SaturateOnIntegerOverflow=on
  Product : Product  SaturateOnIntegerOverflow=on  OutDataTypeStr=Inherit: Same as first input
  Product1 : Product  SaturateOnIntegerOverflow=on  OutDataTypeStr=Inherit: Same as first input
  Product2 : Product  Inputs=***/  SaturateOnIntegerOverflow=on  OutDataTypeStr=Inherit: Same as first input
  Sum1 : Sum  SaturateOnIntegerOverflow=on
  Sum2 : Sum  SaturateOnIntegerOverflow=on
  Switch : Switch  Criteria=u2 ~= 0  SaturateOnIntegerOverflow=on
  mx2 : Outport
  wires:
  Alpha/1 -> Math Function/1, Gain1/1
  Beta/1 -> Gain/1, Math Function1/1
  Gain/1 -> Product/1
  delta elevator/1 -> Product/2
  Gain1/1 -> Product1/1
  delta rudder/1 -> Product1/2
  Product/1 -> Sum1/2
  Product1/1 -> Sum1/1
  Math Function/1 -> Sum2/1
  Math Function1/1 -> Sum2/2
  Constant5/1 -> Product2/3
  Product2/1 -> mx2/1
  Sum1/1 -> Product2/2
  mxad/1 -> Product2/1
  Sum2/1 -> Switch/2, Switch/1
  Switch/1 -> Product2/4
  Constant1/1 -> Switch/3

== system aeromissile_la/Aeromissile Airframe/Thrust(t)/Subsystem/if |u|<0.1 ==
  in : Inport
  Abs : Abs  SaturateOnIntegerOverflow=on
  Constant : Constant  Value=0
  Switch : Switch  Criteria=u2 > Threshold  Threshold=0.1  SaturateOnIntegerOverflow=on
  out : Outport
  wires:
  in/1 -> Switch/1, Abs/1
  Switch/1 -> out/1
  Constant/1 -> Switch/3
  Abs/1 -> Switch/2

== system aeromissile_la/Aeromissile Airframe/Thrust(t)/Subsystem/if |u|<0.1  ==
  in : Inport
  Abs : Abs  SaturateOnIntegerOverflow=on
  Constant : Constant  Value=0
  Switch : Switch  Criteria=u2 > Threshold  Threshold=0.1  SaturateOnIntegerOverflow=on
  out : Outport
  wires:
  in/1 -> Switch/1, Abs/1
  Switch/1 -> out/1
  Constant/1 -> Switch/3
  Abs/1 -> Switch/2

== system aeromissile_la/Visualisation/VR Sink Animation/Euler to VR Quaternion/.... followed by Yaw ==
  e0 : Inport
  "e1 " : Inport  Port=2
  3x3 cross product : Subsystem  mask(Cross Product){}
      mask help: Calculates the cross product of two 3x1 vectors.
      mask Help:
      | <p>This block calculates the cross product of two 3x1 vectors, ie.</p>
      | 
      | <ul>C(1) = A(2)*B(3) - A(3)*B(2)</ul>
      | <ul>C(2) = A(3)*B(1) - A(1)*B(3)</ul>
      | <ul>C(3) = A(1)*B(2) - A(2)*B(1)</ul>
      | 
      | <p>The block inputs and output contain more than one signal as described below.</p>
      | 
      | <p><H4>Block Vector Input 1 - A</H4>
      | <ul>
      | <li>A(1)</li>
      | <li>A(2)</li>
      | <li>A(3)</li>
      | </ul>
      | </p>
      | 
      | <p><H4>Block Vector Input 2 - B</H4>
      | <ul>
      | <li>B(1)</li>
      | <li>B(2)</li>
      | <li>B(3)</li>
      | </ul>
      | </p>
      | 
      | <p><H4>Block Vector Output - Cross Product (AxB)</H4>
      | <ul>
      | <li>C(1)</li>
      | <li>C(2)</li>
      | <li>C(3)</li>
      | </ul>
      | </p>
      mask Display: disp('Cross\nProduct')
  Demux1 : Demux  Outputs=[3 1]
  Demux2 : Demux  Outputs=[3 1]
  Dot Product : DotProduct  InputSameDT=on  OutDataTypeStr=Inherit: Inherit via internal rule
  Mux1 : Mux  Inputs=2
  Product1 : Product  SaturateOnIntegerOverflow=on  InputSameDT=on  OutDataTypeStr=Inherit: Same as first input
  Product2 : Product  SaturateOnIntegerOverflow=on  InputSameDT=on  OutDataTypeStr=Inherit: Same as first input
  Product3 : Product  SaturateOnIntegerOverflow=on  InputSameDT=on  OutDataTypeStr=Inherit: Same as first input
  Sum : Sum  Inputs=+++  SaturateOnIntegerOverflow=on  InputSameDT=on  OutDataTypeStr=Inherit: Same as first input
  Sum1 : Sum  Inputs=-|+  SaturateOnIntegerOverflow=on  InputSameDT=on  OutDataTypeStr=Inherit: Same as first input
  e3 : Outport
  wires:
  "e1 "/1 -> Demux1/1
  e0/1 -> Demux2/1
  Demux1/2 -> Product1/1, Product3/1
  Demux2/1 -> Product1/2, 3x3 cross product/2(b(1) b(2) b(3)), Dot Product/1
  Demux1/1 -> Product2/1, 3x3 cross product/1(a(1) a(2) a(3)), Dot Product/2
  Demux2/2 -> Product2/2, Product3/2
  3x3 cross product/1(c(1) c(2) c(3)) -> Sum/2
  Product2/1 -> Sum/1
  Product1/1 -> Sum/3
  Sum/1 -> Mux1/1
  Dot Product/1 -> Sum1/1
  Product3/1 -> Sum1/2
  Sum1/1 -> Mux1/2
  Mux1/1 -> e3/1

== system aeromissile_la/Visualisation/VR Sink Animation/Euler to VR Quaternion/Align object  ==
  e0 : Inport
  "e1 " : Inport  Port=2
  3x3 cross product : Subsystem  mask(Cross Product){}
      mask help: Calculates the cross product of two 3x1 vectors.
      mask Help:
      | <p>This block calculates the cross product of two 3x1 vectors, ie.</p>
      | 
      | <ul>C(1) = A(2)*B(3) - A(3)*B(2)</ul>
      | <ul>C(2) = A(3)*B(1) - A(1)*B(3)</ul>
      | <ul>C(3) = A(1)*B(2) - A(2)*B(1)</ul>
      | 
      | <p>The block inputs and output contain more than one signal as described below.</p>
      | 
      | <p><H4>Block Vector Input 1 - A</H4>
      | <ul>
      | <li>A(1)</li>
      | <li>A(2)</li>
      | <li>A(3)</li>
      | </ul>
      | </p>
      | 
      | <p><H4>Block Vector Input 2 - B</H4>
      | <ul>
      | <li>B(1)</li>
      | <li>B(2)</li>
      | <li>B(3)</li>
      | </ul>
      | </p>
      | 
      | <p><H4>Block Vector Output - Cross Product (AxB)</H4>
      | <ul>
      | <li>C(1)</li>
      | <li>C(2)</li>
      | <li>C(3)</li>
      | </ul>
      | </p>
      mask Display: disp('Cross\nProduct')
  Demux1 : Demux  Outputs=[3 1]
  Demux2 : Demux  Outputs=[3 1]
  Dot Product : DotProduct  InputSameDT=on  OutDataTypeStr=Inherit: Inherit via internal rule
  Mux1 : Mux  Inputs=2
  Product1 : Product  SaturateOnIntegerOverflow=on  InputSameDT=on  OutDataTypeStr=Inherit: Same as first input
  Product2 : Product  SaturateOnIntegerOverflow=on  InputSameDT=on  OutDataTypeStr=Inherit: Same as first input
  Product3 : Product  SaturateOnIntegerOverflow=on  InputSameDT=on  OutDataTypeStr=Inherit: Same as first input
  Sum : Sum  Inputs=+++  SaturateOnIntegerOverflow=on  InputSameDT=on  OutDataTypeStr=Inherit: Same as first input
  Sum1 : Sum  Inputs=-|+  SaturateOnIntegerOverflow=on  InputSameDT=on  OutDataTypeStr=Inherit: Same as first input
  e3 : Outport
  wires:
  "e1 "/1 -> Demux1/1
  e0/1 -> Demux2/1
  Demux1/2 -> Product1/1, Product3/1
  Demux2/1 -> Product1/2, 3x3 cross product/2(b(1) b(2) b(3)), Dot Product/1
  Demux1/1 -> Product2/1, 3x3 cross product/1(a(1) a(2) a(3)), Dot Product/2
  Demux2/2 -> Product2/2, Product3/2
  3x3 cross product/1(c(1) c(2) c(3)) -> Sum/2
  Product2/1 -> Sum/1
  Product1/1 -> Sum/3
  Sum/1 -> Mux1/1
  Dot Product/1 -> Sum1/1
  Product3/1 -> Sum1/2
  Sum1/1 -> Mux1/2
  Mux1/1 -> e3/1

== system aeromissile_la/Visualisation/VR Sink Animation/Euler to VR Quaternion/Quaternion Normalisation ==
  e0 : Inport
  1/2 : Gain  Gain=1/2  SaturateOnIntegerOverflow=on  OutDataTypeStr=Inherit: Same as input  ParamDataTypeStr=Inherit: Same as input
  Demux : Demux  Outputs=[3 1]
  Mux : Mux  Inputs=2
  Product : Product  SaturateOnIntegerOverflow=on  InputSameDT=on  OutDataTypeStr=Inherit: Same as first input
  Trigonometric Function : Trigonometry
  Trigonometric Function1 : Trigonometry  Operator=cos
  e0_norm : Outport
  wires:
  Mux/1 -> e0_norm/1
  Trigonometric Function1/1 -> Mux/2
  Product/1 -> Mux/1
  Demux/1 -> Product/1
  Trigonometric Function/1 -> Product/2
  Demux/2 -> 1/2/1
  1/2/1 -> Trigonometric Function1/1, Trigonometric Function/1
  e0/1 -> Demux/1

== system aeromissile_la/Visualisation/VR Sink Animation/Euler to VR Quaternion/Quaternion Normalisation  ==
  e0 : Inport
  1/2 : Gain  Gain=1/2  SaturateOnIntegerOverflow=on  OutDataTypeStr=Inherit: Same as input  ParamDataTypeStr=Inherit: Same as input
  Demux : Demux  Outputs=[3 1]
  Mux : Mux  Inputs=2
  Product : Product  SaturateOnIntegerOverflow=on  InputSameDT=on  OutDataTypeStr=Inherit: Same as first input
  Trigonometric Function : Trigonometry
  Trigonometric Function1 : Trigonometry  Operator=cos
  e0_norm : Outport
  wires:
  e0/1 -> Demux/1
  1/2/1 -> Trigonometric Function/1, Trigonometric Function1/1
  Demux/2 -> 1/2/1
  Trigonometric Function/1 -> Product/2
  Demux/1 -> Product/1
  Product/1 -> Mux/1
  Trigonometric Function1/1 -> Mux/2
  Mux/1 -> e0_norm/1

== system aeromissile_la/Visualisation/VR Sink Animation/Euler to VR Quaternion/Quaternion Normalisation   ==
  e0 : Inport
  1/2 : Gain  Gain=1/2  SaturateOnIntegerOverflow=on  OutDataTypeStr=Inherit: Same as input  ParamDataTypeStr=Inherit: Same as input
  Demux : Demux  Outputs=[3 1]
  Mux : Mux  Inputs=2
  Product : Product  SaturateOnIntegerOverflow=on  InputSameDT=on  OutDataTypeStr=Inherit: Same as first input
  Trigonometric Function : Trigonometry
  Trigonometric Function1 : Trigonometry  Operator=cos
  e0_norm : Outport
  wires:
  e0/1 -> Demux/1
  1/2/1 -> Trigonometric Function/1, Trigonometric Function1/1
  Demux/2 -> 1/2/1
  Trigonometric Function/1 -> Product/2
  Demux/1 -> Product/1
  Product/1 -> Mux/1
  Trigonometric Function1/1 -> Mux/2
  Mux/1 -> e0_norm/1

== system aeromissile_la/Visualisation/VR Sink Animation/Euler to VR Quaternion/Quaternion Normalisation    ==
  e0 : Inport
  1/2 : Gain  Gain=1/2  SaturateOnIntegerOverflow=on  OutDataTypeStr=Inherit: Same as input  ParamDataTypeStr=Inherit: Same as input
  Demux : Demux  Outputs=[3 1]
  Mux : Mux  Inputs=2
  Product : Product  SaturateOnIntegerOverflow=on  InputSameDT=on  OutDataTypeStr=Inherit: Same as first input
  Trigonometric Function : Trigonometry
  Trigonometric Function1 : Trigonometry  Operator=cos
  e0_norm : Outport
  wires:
  Mux/1 -> e0_norm/1
  Trigonometric Function1/1 -> Mux/2
  Product/1 -> Mux/1
  Demux/1 -> Product/1
  Trigonometric Function/1 -> Product/2
  Demux/2 -> 1/2/1
  1/2/1 -> Trigonometric Function1/1, Trigonometric Function/1
  e0/1 -> Demux/1

== system aeromissile_la/Visualisation/VR Sink Animation/Euler to VR Quaternion/Quaternion Vector ==
  e0 : Inport
  2 : Gain  Gain=2  SaturateOnIntegerOverflow=on  OutDataTypeStr=Inherit: Same as input  ParamDataTypeStr=Inherit: Same as input
  Demux : Demux  Outputs=[3 1]
  Mux : Mux  Inputs=2
  Product : Product  Inputs=*/  SaturateOnIntegerOverflow=on  InputSameDT=on  OutDataTypeStr=Inherit: Same as first input
  Trigonometric Function : Trigonometry
  Trigonometric Function2 : Trigonometry  Operator=acos
  e0_norm : Outport
  wires:
  Mux/1 -> e0_norm/1
  Product/1 -> Mux/1
  2/1 -> Mux/2
  Trigonometric Function/1 -> Product/2
  Demux/1 -> Product/1
  Trigonometric Function2/1 -> Trigonometric Function/1, 2/1
  Demux/2 -> Trigonometric Function2/1
  e0/1 -> Demux/1

== system aeromissile_la/Visualisation/VR Sink Animation/Euler to VR Quaternion/Roll followed by Pitch ==
  e0 : Inport
  "e1 " : Inport  Port=2
  3x3 cross product : Subsystem  mask(Cross Product){}
      mask help: Calculates the cross product of two 3x1 vectors.
      mask Help:
      | <p>This block calculates the cross product of two 3x1 vectors, ie.</p>
      | 
      | <ul>C(1) = A(2)*B(3) - A(3)*B(2)</ul>
      | <ul>C(2) = A(3)*B(1) - A(1)*B(3)</ul>
      | <ul>C(3) = A(1)*B(2) - A(2)*B(1)</ul>
      | 
      | <p>The block inputs and output contain more than one signal as described below.</p>
      | 
      | <p><H4>Block Vector Input 1 - A</H4>
      | <ul>
      | <li>A(1)</li>
      | <li>A(2)</li>
      | <li>A(3)</li>
      | </ul>
      | </p>
      | 
      | <p><H4>Block Vector Input 2 - B</H4>
      | <ul>
      | <li>B(1)</li>
      | <li>B(2)</li>
      | <li>B(3)</li>
      | </ul>
      | </p>
      | 
      | <p><H4>Block Vector Output - Cross Product (AxB)</H4>
      | <ul>
      | <li>C(1)</li>
      | <li>C(2)</li>
      | <li>C(3)</li>
      | </ul>
      | </p>
      mask Display: disp('Cross\nProduct')
  Demux1 : Demux  Outputs=[3 1]
  Demux2 : Demux  Outputs=[3 1]
  Dot Product : DotProduct  InputSameDT=on  OutDataTypeStr=Inherit: Inherit via internal rule
  Mux1 : Mux  Inputs=2
  Product1 : Product  SaturateOnIntegerOverflow=on  InputSameDT=on  OutDataTypeStr=Inherit: Same as first input
  Product2 : Product  SaturateOnIntegerOverflow=on  InputSameDT=on  OutDataTypeStr=Inherit: Same as first input
  Product3 : Product  SaturateOnIntegerOverflow=on  InputSameDT=on  OutDataTypeStr=Inherit: Same as first input
  Sum : Sum  Inputs=+++  SaturateOnIntegerOverflow=on  InputSameDT=on  OutDataTypeStr=Inherit: Same as first input
  Sum1 : Sum  Inputs=-|+  SaturateOnIntegerOverflow=on  InputSameDT=on  OutDataTypeStr=Inherit: Same as first input
  e3 : Outport
  wires:
  Mux1/1 -> e3/1
  Sum1/1 -> Mux1/2
  Product3/1 -> Sum1/2
  Dot Product/1 -> Sum1/1
  Sum/1 -> Mux1/1
  Product1/1 -> Sum/3
  Product2/1 -> Sum/1
  3x3 cross product/1(c(1) c(2) c(3)) -> Sum/2
  Demux2/2 -> Product3/2, Product2/2
  Demux1/1 -> Dot Product/2, 3x3 cross product/1(a(1) a(2) a(3)), Product2/1
  Demux2/1 -> Dot Product/1, 3x3 cross product/2(b(1) b(2) b(3)), Product1/2
  Demux1/2 -> Product3/1, Product1/1
  e0/1 -> Demux2/1
  "e1 "/1 -> Demux1/1

== system aeromissile_la/Aeromissile Airframe/6DoF Ru (Euler Angles) Mvar/inertia^(-1)x(M-C)/inertia(t)^-1/inertia(t) ==
  Constant : Constant  Value=inertia_0
  Constant1 : Constant  Value=inertia
  Constant2 : Constant  Value=q
  Constant3 : Constant  Value=massf
  Product : Product  Inputs=**/  SaturateOnIntegerOverflow=on  OutDataTypeStr=Inherit: Same as first input
  Product1 : Product  SaturateOnIntegerOverflow=on  OutDataTypeStr=Inherit: Same as first input
  Scope : Scope
  Sum : Sum  Inputs=|+-  SaturateOnIntegerOverflow=on
  Sum1 : Sum  Inputs=|+-  SaturateOnIntegerOverflow=on
  Sum3 : Sum  Inputs=|+-  SaturateOnIntegerOverflow=on
  Switch : Switch  Criteria=u2 > Threshold  SaturateOnIntegerOverflow=on
  inertia(t) : Outport
  wires:
  Constant/1 -> Sum1/1, Sum/1
  Constant1/1 -> Sum1/2, Switch/3
  Sum1/1 -> Product/1
  Product/1 -> Sum/2
  Switch/1 -> inertia(t)/1, Scope/1
  Sum/1 -> Switch/1
  Constant2/1 -> Product1/1
  [tE] -> Product1/2
  Sum3/1 -> Switch/2
  Product1/1 -> Product/2, Sum3/2
  Constant3/1 -> Product/3, Sum3/1

== system aeromissile_la/Visualisation/VR Sink Animation/Euler to VR Quaternion/.... followed by Yaw/3x3 cross product ==
  a(1) a(2) a(3) : Inport
  b(1) b(2) b(3) : Inport  Port=2
  Product : Product  SaturateOnIntegerOverflow=on  InputSameDT=on  OutDataTypeStr=Inherit: Same as first input
  Product1 : Product  SaturateOnIntegerOverflow=on  InputSameDT=on  OutDataTypeStr=Inherit: Same as first input
  Selector : Selector  InputPortWidth=3  IndexOptions=Index vector (dialog)  Indices=[2 3 1]  OutputSizes=1
  Selector1 : Selector  InputPortWidth=3  IndexOptions=Index vector (dialog)  Indices=[3 1 2]  OutputSizes=1
  Selector2 : Selector  InputPortWidth=3  IndexOptions=Index vector (dialog)  Indices=[2 3 1]  OutputSizes=1
  Selector3 : Selector  InputPortWidth=3  IndexOptions=Index vector (dialog)  Indices=[3 1 2]  OutputSizes=1
  Sum : Sum  Inputs=+|-  SaturateOnIntegerOverflow=on  InputSameDT=on  OutDataTypeStr=Inherit: Same as first input
  c(1) c(2) c(3) : Outport  InitialOutput=0
  wires:
  Selector3/1 -> Product1/1
  Selector2/1 -> Product1/2
  Product1/1 -> Sum/2
  Selector1/1 -> Product/2
  Product/1 -> Sum/1
  a(1) a(2) a(3)/1 -> Selector3/1, Selector/1
  Selector/1 -> Product/1
  b(1) b(2) b(3)/1 -> Selector2/1, Selector1/1
  Sum/1 -> c(1) c(2) c(3)/1

== system aeromissile_la/Visualisation/VR Sink Animation/Euler to VR Quaternion/Align object /3x3 cross product ==
  a(1) a(2) a(3) : Inport
  b(1) b(2) b(3) : Inport  Port=2
  Product : Product  SaturateOnIntegerOverflow=on  InputSameDT=on  OutDataTypeStr=Inherit: Same as first input
  Product1 : Product  SaturateOnIntegerOverflow=on  InputSameDT=on  OutDataTypeStr=Inherit: Same as first input
  Selector : Selector  InputPortWidth=3  IndexOptions=Index vector (dialog)  Indices=[2 3 1]  OutputSizes=1
  Selector1 : Selector  InputPortWidth=3  IndexOptions=Index vector (dialog)  Indices=[3 1 2]  OutputSizes=1
  Selector2 : Selector  InputPortWidth=3  IndexOptions=Index vector (dialog)  Indices=[2 3 1]  OutputSizes=1
  Selector3 : Selector  InputPortWidth=3  IndexOptions=Index vector (dialog)  Indices=[3 1 2]  OutputSizes=1
  Sum : Sum  Inputs=+|-  SaturateOnIntegerOverflow=on  InputSameDT=on  OutDataTypeStr=Inherit: Same as first input
  c(1) c(2) c(3) : Outport  InitialOutput=0
  wires:
  Selector3/1 -> Product1/1
  Selector2/1 -> Product1/2
  Product1/1 -> Sum/2
  Selector1/1 -> Product/2
  Product/1 -> Sum/1
  a(1) a(2) a(3)/1 -> Selector3/1, Selector/1
  Selector/1 -> Product/1
  b(1) b(2) b(3)/1 -> Selector2/1, Selector1/1
  Sum/1 -> c(1) c(2) c(3)/1

== system aeromissile_la/Visualisation/VR Sink Animation/Euler to VR Quaternion/Roll followed by Pitch/3x3 cross product ==
  a(1) a(2) a(3) : Inport
  b(1) b(2) b(3) : Inport  Port=2
  Product : Product  SaturateOnIntegerOverflow=on  InputSameDT=on  OutDataTypeStr=Inherit: Same as first input
  Product1 : Product  SaturateOnIntegerOverflow=on  InputSameDT=on  OutDataTypeStr=Inherit: Same as first input
  Selector : Selector  InputPortWidth=3  IndexOptions=Index vector (dialog)  Indices=[2 3 1]  OutputSizes=1
  Selector1 : Selector  InputPortWidth=3  IndexOptions=Index vector (dialog)  Indices=[3 1 2]  OutputSizes=1
  Selector2 : Selector  InputPortWidth=3  IndexOptions=Index vector (dialog)  Indices=[2 3 1]  OutputSizes=1
  Selector3 : Selector  InputPortWidth=3  IndexOptions=Index vector (dialog)  Indices=[3 1 2]  OutputSizes=1
  Sum : Sum  Inputs=+|-  SaturateOnIntegerOverflow=on  InputSameDT=on  OutDataTypeStr=Inherit: Same as first input
  c(1) c(2) c(3) : Outport  InitialOutput=0
  wires:
  Sum/1 -> c(1) c(2) c(3)/1
  b(1) b(2) b(3)/1 -> Selector1/1, Selector2/1
  Selector/1 -> Product/1
  a(1) a(2) a(3)/1 -> Selector/1, Selector3/1
  Product/1 -> Sum/1
  Selector1/1 -> Product/2
  Product1/1 -> Sum/2
  Selector2/1 -> Product1/2
  Selector3/1 -> Product1/1
